simulink model "gm_rec_i2s"  (R2023b)
settings: Solver=VariableStepAuto  StartTime=0.0  StopTime=20  RelTol=1e-3
undefined symbols (not defined in the file or in its folder): cnt1_LRCLK, cnt2_SCLK
libraries: hdlsllib x4
(part 1 of 3)
settings Model: Creator=31651  LastModifiedBy=31651
settings DataIOCC: SignalLogging=off
settings OptimizationCC: BlockReduction=off  ConditionallyExecuteInputs=off  DefaultParameterBehavior=Inlined
settings DebuggingCC: AlgebraicLoopMsg=error  InheritedTsInSrcMsg=none
settings HardwareCC: ProdBitPerPointer=32  ProdBitPerSizeT=32  ProdBitPerPtrDiffT=32  ProdLargestAtomicFloat=None  ProdIntDivRoundTo=Undefined  ProdEndianess=Unspecified  ProdWordSize=32  ProdHWDeviceType=ASIC/FPGA->ASIC/FPGA  TargetBitPerPointer=64  TargetBitPerSizeT=64  TargetBitPerPtrDiffT=64  TargetLongLongMode=on  TargetIntDivRoundTo=Zero  TargetEndianess=LittleEndian  TargetWordSize=64  TargetHWDeviceType=Custom Processor->MATLAB Host Computer  ProdEqTarget=off

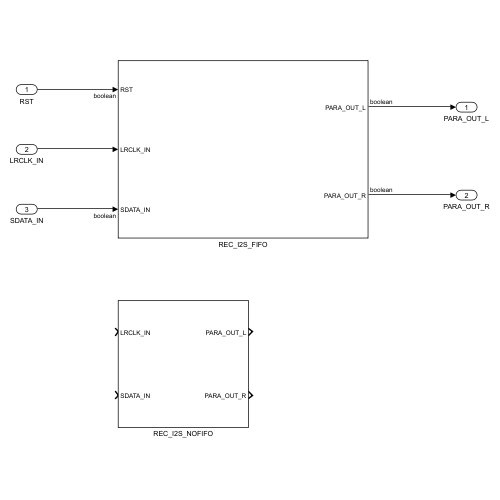
[thumbnail: Simulink's stored preview of the top-level diagram]
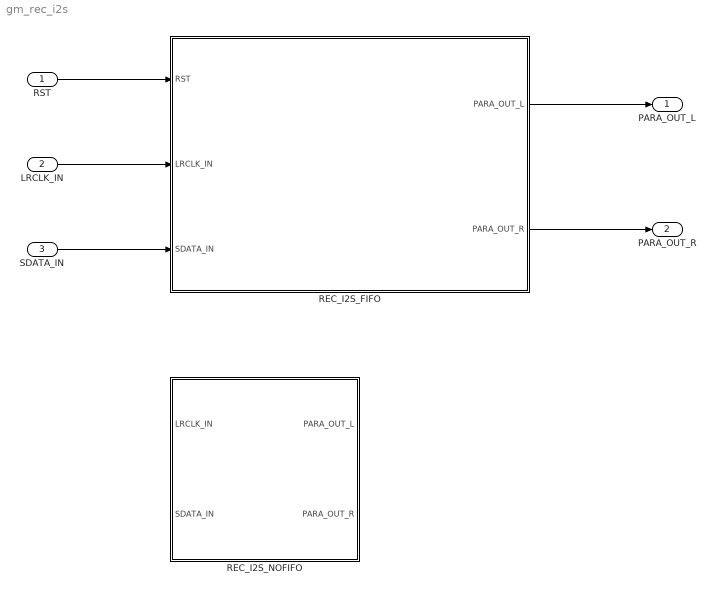
== system gm_rec_i2s ==
  RST : Inport
  LRCLK_IN : Inport  Port=2
  SDATA_IN : Inport  Port=3
  REC_I2S_FIFO : Subsystem
  REC_I2S_NOFIFO : Subsystem
  PARA_OUT_L : Outport
  PARA_OUT_R : Outport  Port=2
  wires:
  REC_I2S_FIFO/2(PARA_OUT_R) -> PARA_OUT_R/1
  REC_I2S_FIFO/1(PARA_OUT_L) -> PARA_OUT_L/1
  SDATA_IN/1 -> REC_I2S_FIFO/3(SDATA_IN)
  LRCLK_IN/1 -> REC_I2S_FIFO/2(LRCLK_IN)
  RST/1 -> REC_I2S_FIFO/1(RST)

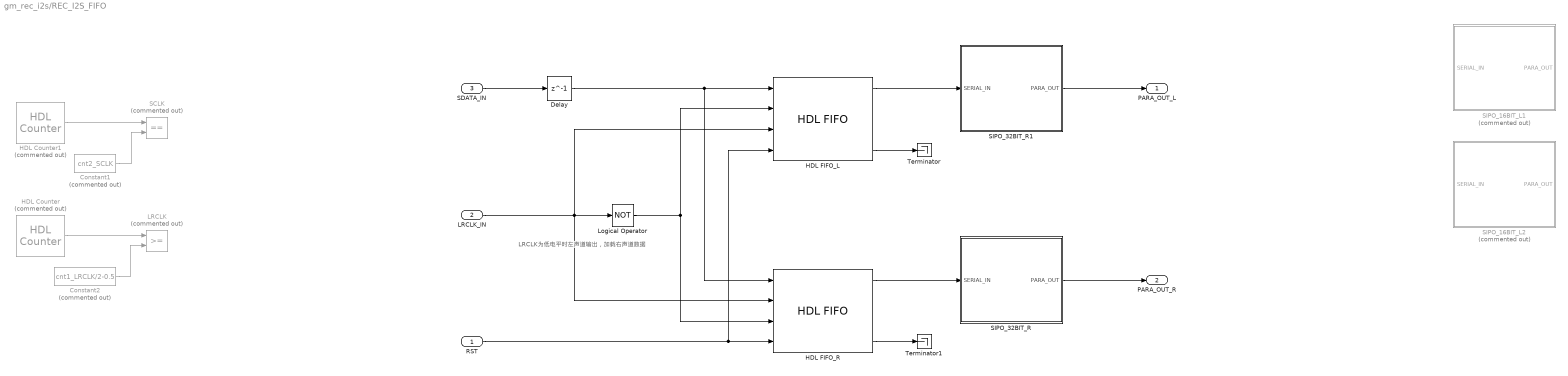
== system gm_rec_i2s/REC_I2S_FIFO ==
  note: LRCLK为低电平时左声道输出，加载右声道数据
  RST : Inport  OutDataTypeStr=boolean
  LRCLK_IN : Inport  Port=2
  SDATA_IN : Inport  Port=3  OutDataTypeStr=boolean
  Constant1 : Constant  Commented=on  Value=cnt2_SCLK  OutDataTypeStr=uint16
  Constant2 : Constant  Commented=on  Value=cnt1_LRCLK/2-0.5  OutDataTypeStr=uint16
  Delay : Delay  DelayLength=1  InitialCondition=0  SampleTime=1
  HDL Counter : hdlsllib/Sources/HDL Counter  Commented=on  CountType=Count limited  CountInit=0  CountStep=1  CountMax=cnt1_LRCLK  CountFromType=Initial value  CountFrom=0  CountResetPort=off  CountLoadPort=off  CountEnbPort=on  CountDirPort=off  CountHitOutputPort=off  CountDataType=Unsigned  CountWordLen=16  CountFracLen=0  CountSampTime=1
  HDL Counter1 : hdlsllib/Sources/HDL Counter  Commented=on  CountType=Count limited  CountInit=0  CountStep=1  CountMax=cnt2_SCLK  CountFromType=Initial value  CountFrom=0  CountResetPort=off  CountLoadPort=off  CountEnbPort=on  CountDirPort=off  CountHitOutputPort=off  CountDataType=Unsigned  CountWordLen=16  CountFracLen=0  CountSampTime=1
  HDL FIFO_L : hdlsllib/HDL RAMs/HDL FIFO  fifo_size=32  mode=Classic  ratio=1  push_msg=Warning  pop_msg=Warning  show_empty=on  show_full=on  show_num=on  LabelModeActiveChoice_Mode=Classic  rst_port=on
  HDL FIFO_R : hdlsllib/HDL RAMs/HDL FIFO  fifo_size=32  mode=Classic  ratio=1  push_msg=Warning  pop_msg=Warning  show_empty=on  show_full=on  show_num=on  LabelModeActiveChoice_Mode=Classic  rst_port=on
  LRCLK : RelationalOperator  Commented=on  OutDataTypeStr=boolean  InputSameDT=off
  Logical Operator : Logic  Operator=NOT  AllPortsSameDT=off  OutDataTypeStr=boolean
  SCLK : RelationalOperator  Commented=on  Operator===  OutDataTypeStr=boolean  InputSameDT=off
  SIPO_16BIT_L1 : Subsystem  Commented=on
  SIPO_16BIT_L2 : Subsystem  Commented=on
  SIPO_32BIT_R : Subsystem
  SIPO_32BIT_R1 : Subsystem
  Terminator : Terminator
  Terminator1 : Terminator
  PARA_OUT_L : Outport  OutDataTypeStr=boolean
  PARA_OUT_R : Outport  Port=2  OutDataTypeStr=boolean
  wires:
  HDL FIFO_L/1 -> SIPO_32BIT_R1/1(SERIAL_IN)
  HDL FIFO_R/1 -> SIPO_32BIT_R/1(SERIAL_IN)
  SIPO_32BIT_R/1(PARA_OUT) -> PARA_OUT_R/1
  SIPO_32BIT_R1/1(PARA_OUT) -> PARA_OUT_L/1
  RST/1 -> HDL FIFO_R/4, HDL FIFO_L/4
  Delay/1 -> HDL FIFO_L/1, HDL FIFO_R/1
  SDATA_IN/1 -> Delay/1
  HDL FIFO_R/4 -> Terminator1/1
  HDL FIFO_L/4 -> Terminator/1
  LRCLK_IN/1 -> Logical Operator/1, HDL FIFO_L/3, HDL FIFO_R/2
  Constant2/1 -> LRCLK/2
  Constant1/1 -> SCLK/2
  HDL Counter/1 -> LRCLK/1
  Logical Operator/1 -> HDL FIFO_R/3, HDL FIFO_L/2
  HDL Counter1/1 -> SCLK/1

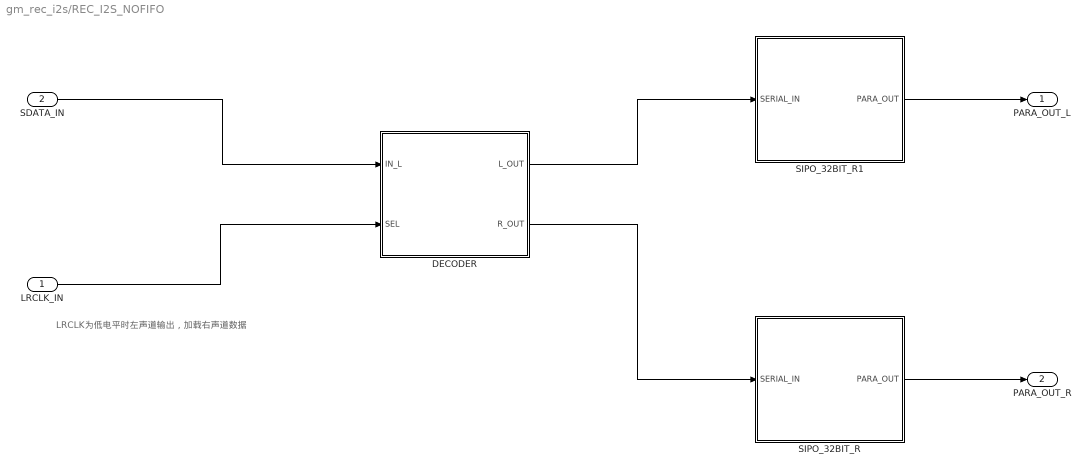
== system gm_rec_i2s/REC_I2S_NOFIFO ==
  note: LRCLK为低电平时左声道输出，加载右声道数据
  LRCLK_IN : Inport
  SDATA_IN : Inport  Port=2  OutDataTypeStr=boolean
  DECODER : Subsystem
  SIPO_32BIT_R : Subsystem
  SIPO_32BIT_R1 : Subsystem
  PARA_OUT_L : Outport  OutDataTypeStr=boolean
  PARA_OUT_R : Outport  Port=2  OutDataTypeStr=boolean
  wires:
  DECODER/2(R_OUT) -> SIPO_32BIT_R/1(SERIAL_IN)
  DECODER/1(L_OUT) -> SIPO_32BIT_R1/1(SERIAL_IN)
  LRCLK_IN/1 -> DECODER/2(SEL)
  SIPO_32BIT_R/1(PARA_OUT) -> PARA_OUT_R/1
  SDATA_IN/1 -> DECODER/1(IN_L)
  SIPO_32BIT_R1/1(PARA_OUT) -> PARA_OUT_L/1

== system gm_rec_i2s/REC_I2S_FIFO/SIPO_16BIT_L1 ==
  SERIAL_IN : Inport  OutDataTypeStr=boolean
  Merge : Merge
  SIPO_8BIT : Subsystem
  SIPO_8BIT1 : Subsystem
  Terminator : Terminator
  PARA_OUT : Outport  VectorParamsAs1DForOutWhenUnconnected=off
  wires:
  Merge/1 -> PARA_OUT/1
  SIPO_8BIT1/2(SERIAL_OUT) -> Terminator/1
  SIPO_8BIT1/1(PARA_OUT) -> Merge/1
  SIPO_8BIT/1(PARA_OUT) -> Merge/2
  SIPO_8BIT/2(SERIAL_OUT) -> SIPO_8BIT1/1(SERIAL_IN)
  SERIAL_IN/1 -> SIPO_8BIT/1(SERIAL_IN)

== system gm_rec_i2s/REC_I2S_FIFO/SIPO_16BIT_L2 ==
  SERIAL_IN : Inport  OutDataTypeStr=boolean
  Merge : Merge
  SIPO_8BIT : Subsystem
  SIPO_8BIT1 : Subsystem
  Terminator : Terminator
  PARA_OUT : Outport  VectorParamsAs1DForOutWhenUnconnected=off
  wires:
  Merge/1 -> PARA_OUT/1
  SIPO_8BIT1/2(SERIAL_OUT) -> Terminator/1
  SIPO_8BIT1/1(PARA_OUT) -> Merge/1
  SIPO_8BIT/1(PARA_OUT) -> Merge/2
  SIPO_8BIT/2(SERIAL_OUT) -> SIPO_8BIT1/1(SERIAL_IN)
  SERIAL_IN/1 -> SIPO_8BIT/1(SERIAL_IN)

== system gm_rec_i2s/REC_I2S_FIFO/SIPO_32BIT_R ==
  SERIAL_IN : Inport  OutDataTypeStr=boolean
  Subsystem : Subsystem
  PARA_OUT : Outport  OutDataTypeStr=boolean  VectorParamsAs1DForOutWhenUnconnected=off
  wires:
  Subsystem/1(PARA_OUT_32BIT) -> PARA_OUT/1
  SERIAL_IN/1 -> Subsystem/1(SERIAL_IN)

== system gm_rec_i2s/REC_I2S_FIFO/SIPO_32BIT_R1 ==
  SERIAL_IN : Inport  OutDataTypeStr=boolean
  Subsystem : Subsystem
  PARA_OUT : Outport  OutDataTypeStr=boolean  VectorParamsAs1DForOutWhenUnconnected=off
  wires:
  Subsystem/1(PARA_OUT_32BIT) -> PARA_OUT/1
  SERIAL_IN/1 -> Subsystem/1(SERIAL_IN)

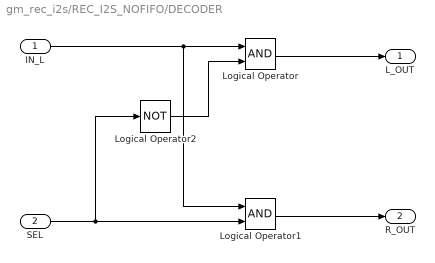
== system gm_rec_i2s/REC_I2S_NOFIFO/DECODER ==
  IN_L : Inport  OutDataTypeStr=boolean
  SEL : Inport  Port=2  OutDataTypeStr=boolean
  Logical Operator : Logic  AllPortsSameDT=off  OutDataTypeStr=boolean
  Logical Operator1 : Logic  AllPortsSameDT=off  OutDataTypeStr=boolean
  Logical Operator2 : Logic  Operator=NOT  AllPortsSameDT=off  OutDataTypeStr=boolean
  L_OUT : Outport  VectorParamsAs1DForOutWhenUnconnected=off
  R_OUT : Outport  Port=2  VectorParamsAs1DForOutWhenUnconnected=off
  wires:
  Logical Operator1/1 -> R_OUT/1
  Logical Operator/1 -> L_OUT/1
  IN_L/1 -> Logical Operator/1, Logical Operator1/1
  Logical Operator2/1 -> Logical Operator/2
  SEL/1 -> Logical Operator2/1, Logical Operator1/2

== system gm_rec_i2s/REC_I2S_NOFIFO/SIPO_32BIT_R ==
  SERIAL_IN : Inport  OutDataTypeStr=boolean
  Subsystem : Subsystem
  PARA_OUT : Outport  OutDataTypeStr=boolean  VectorParamsAs1DForOutWhenUnconnected=off
  wires:
  Subsystem/1(PARA_OUT_32BIT) -> PARA_OUT/1
  SERIAL_IN/1 -> Subsystem/1(SERIAL_IN)

== system gm_rec_i2s/REC_I2S_NOFIFO/SIPO_32BIT_R1 ==
  SERIAL_IN : Inport  OutDataTypeStr=boolean
  Subsystem : Subsystem
  PARA_OUT : Outport  OutDataTypeStr=boolean  VectorParamsAs1DForOutWhenUnconnected=off
  wires:
  Subsystem/1(PARA_OUT_32BIT) -> PARA_OUT/1
  SERIAL_IN/1 -> Subsystem/1(SERIAL_IN)

== system gm_rec_i2s/REC_I2S_FIFO/SIPO_16BIT_L1/SIPO_8BIT ==
  SERIAL_IN : Inport  OutDataTypeStr=boolean
  Merge : Merge
  SIPO_4BIT : Subsystem
  SIPO_4BIT1 : Subsystem
  PARA_OUT : Outport  VectorParamsAs1DForOutWhenUnconnected=off
  SERIAL_OUT : Outport  Port=2  VectorParamsAs1DForOutWhenUnconnected=off
  wires:
  SERIAL_IN/1 -> SIPO_4BIT/1(SERIAL_IN)
  SIPO_4BIT1/2(SERIAL_OUT) -> SERIAL_OUT/1
  SIPO_4BIT1/1(PARA_OUT) -> Merge/1
  SIPO_4BIT/2(SERIAL_OUT) -> SIPO_4BIT1/1(SERIAL_IN)
  Merge/1 -> PARA_OUT/1
  SIPO_4BIT/1(PARA_OUT) -> Merge/2

== system gm_rec_i2s/REC_I2S_FIFO/SIPO_16BIT_L1/SIPO_8BIT1 ==
  SERIAL_IN : Inport  OutDataTypeStr=boolean
  Merge : Merge
  SIPO_4BIT : Subsystem
  SIPO_4BIT1 : Subsystem
  PARA_OUT : Outport  VectorParamsAs1DForOutWhenUnconnected=off
  SERIAL_OUT : Outport  Port=2  VectorParamsAs1DForOutWhenUnconnected=off
  wires:
  SERIAL_IN/1 -> SIPO_4BIT/1(SERIAL_IN)
  SIPO_4BIT1/2(SERIAL_OUT) -> SERIAL_OUT/1
  SIPO_4BIT1/1(PARA_OUT) -> Merge/1
  SIPO_4BIT/2(SERIAL_OUT) -> SIPO_4BIT1/1(SERIAL_IN)
  Merge/1 -> PARA_OUT/1
  SIPO_4BIT/1(PARA_OUT) -> Merge/2

== system gm_rec_i2s/REC_I2S_FIFO/SIPO_16BIT_L2/SIPO_8BIT ==
  SERIAL_IN : Inport  OutDataTypeStr=boolean
  Merge : Merge
  SIPO_4BIT : Subsystem
  SIPO_4BIT1 : Subsystem
  PARA_OUT : Outport  VectorParamsAs1DForOutWhenUnconnected=off
  SERIAL_OUT : Outport  Port=2  VectorParamsAs1DForOutWhenUnconnected=off
  wires:
  SERIAL_IN/1 -> SIPO_4BIT/1(SERIAL_IN)
  SIPO_4BIT1/2(SERIAL_OUT) -> SERIAL_OUT/1
  SIPO_4BIT1/1(PARA_OUT) -> Merge/1
  SIPO_4BIT/2(SERIAL_OUT) -> SIPO_4BIT1/1(SERIAL_IN)
  Merge/1 -> PARA_OUT/1
  SIPO_4BIT/1(PARA_OUT) -> Merge/2

== system gm_rec_i2s/REC_I2S_FIFO/SIPO_16BIT_L2/SIPO_8BIT1 ==
  SERIAL_IN : Inport  OutDataTypeStr=boolean
  Merge : Merge
  SIPO_4BIT : Subsystem
  SIPO_4BIT1 : Subsystem
  PARA_OUT : Outport  VectorParamsAs1DForOutWhenUnconnected=off
  SERIAL_OUT : Outport  Port=2  VectorParamsAs1DForOutWhenUnconnected=off
  wires:
  SERIAL_IN/1 -> SIPO_4BIT/1(SERIAL_IN)
  SIPO_4BIT1/2(SERIAL_OUT) -> SERIAL_OUT/1
  SIPO_4BIT1/1(PARA_OUT) -> Merge/1
  SIPO_4BIT/2(SERIAL_OUT) -> SIPO_4BIT1/1(SERIAL_IN)
  Merge/1 -> PARA_OUT/1
  SIPO_4BIT/1(PARA_OUT) -> Merge/2

== system gm_rec_i2s/REC_I2S_FIFO/SIPO_32BIT_R/Subsystem ==
  SERIAL_IN : Inport  OutDataTypeStr=boolean
  SIPO_16BIT : Subsystem
  SIPO_16BIT1 : Subsystem
  Terminator : Terminator
  Vector Concatenate : Concatenate
  PARA_OUT_32BIT : Outport
  wires:
  Vector Concatenate/1 -> PARA_OUT_32BIT/1
  SIPO_16BIT1/2(SERIAL_OUT) -> Terminator/1
  SIPO_16BIT1/1(PARA_OUT) -> Vector Concatenate/1
  SIPO_16BIT/1(PARA_OUT) -> Vector Concatenate/2
  SIPO_16BIT/2(SERIAL_OUT) -> SIPO_16BIT1/1(SERIAL_IN)
  SERIAL_IN/1 -> SIPO_16BIT/1(SERIAL_IN)

== system gm_rec_i2s/REC_I2S_FIFO/SIPO_32BIT_R1/Subsystem ==
  SERIAL_IN : Inport  OutDataTypeStr=boolean
  SIPO_16BIT : Subsystem
  SIPO_16BIT1 : Subsystem
  Terminator : Terminator
  Vector Concatenate : Concatenate
  PARA_OUT_32BIT : Outport
  wires:
  Vector Concatenate/1 -> PARA_OUT_32BIT/1
  SIPO_16BIT1/2(SERIAL_OUT) -> Terminator/1
  SIPO_16BIT1/1(PARA_OUT) -> Vector Concatenate/1
  SIPO_16BIT/1(PARA_OUT) -> Vector Concatenate/2
  SIPO_16BIT/2(SERIAL_OUT) -> SIPO_16BIT1/1(SERIAL_IN)
  SERIAL_IN/1 -> SIPO_16BIT/1(SERIAL_IN)

== system gm_rec_i2s/REC_I2S_NOFIFO/SIPO_32BIT_R/Subsystem ==
  SERIAL_IN : Inport  OutDataTypeStr=boolean
  SIPO_16BIT : Subsystem
  SIPO_16BIT1 : Subsystem
  Terminator : Terminator
  Vector Concatenate : Concatenate
  PARA_OUT_32BIT : Outport
  wires:
  Vector Concatenate/1 -> PARA_OUT_32BIT/1
  SIPO_16BIT1/2(SERIAL_OUT) -> Terminator/1
  SIPO_16BIT1/1(PARA_OUT) -> Vector Concatenate/1
  SIPO_16BIT/1(PARA_OUT) -> Vector Concatenate/2
  SIPO_16BIT/2(SERIAL_OUT) -> SIPO_16BIT1/1(SERIAL_IN)
  SERIAL_IN/1 -> SIPO_16BIT/1(SERIAL_IN)

== system gm_rec_i2s/REC_I2S_NOFIFO/SIPO_32BIT_R1/Subsystem ==
  SERIAL_IN : Inport  OutDataTypeStr=boolean
  SIPO_16BIT : Subsystem
  SIPO_16BIT1 : Subsystem
  Terminator : Terminator
  Vector Concatenate : Concatenate
  PARA_OUT_32BIT : Outport
  wires:
  Vector Concatenate/1 -> PARA_OUT_32BIT/1
  SIPO_16BIT1/2(SERIAL_OUT) -> Terminator/1
  SIPO_16BIT1/1(PARA_OUT) -> Vector Concatenate/1
  SIPO_16BIT/1(PARA_OUT) -> Vector Concatenate/2
  SIPO_16BIT/2(SERIAL_OUT) -> SIPO_16BIT1/1(SERIAL_IN)
  SERIAL_IN/1 -> SIPO_16BIT/1(SERIAL_IN)

== system gm_rec_i2s/REC_I2S_FIFO/SIPO_16BIT_L1/SIPO_8BIT/SIPO_4BIT ==
  SERIAL_IN : Inport
  2BIT_SIPO : Subsystem
  2BIT_SIPO1 : Subsystem
  Merge : Merge
  PARA_OUT : Outport  VectorParamsAs1DForOutWhenUnconnected=off
  SERIAL_OUT : Outport  Port=2  VectorParamsAs1DForOutWhenUnconnected=off
  wires:
  2BIT_SIPO/2(SERIAL_OUT) -> 2BIT_SIPO1/1(SERIAL_IN)
  2BIT_SIPO1/1(PARA_OUT) -> Merge/1
  2BIT_SIPO/1(PARA_OUT) -> Merge/2
  Merge/1 -> PARA_OUT/1
  2BIT_SIPO1/2(SERIAL_OUT) -> SERIAL_OUT/1
  SERIAL_IN/1 -> 2BIT_SIPO/1(SERIAL_IN)

== system gm_rec_i2s/REC_I2S_FIFO/SIPO_16BIT_L1/SIPO_8BIT/SIPO_4BIT1 ==
  SERIAL_IN : Inport
  2BIT_SIPO : Subsystem
  2BIT_SIPO1 : Subsystem
  Merge : Merge
  PARA_OUT : Outport  VectorParamsAs1DForOutWhenUnconnected=off
  SERIAL_OUT : Outport  Port=2  VectorParamsAs1DForOutWhenUnconnected=off
  wires:
  2BIT_SIPO/2(SERIAL_OUT) -> 2BIT_SIPO1/1(SERIAL_IN)
  2BIT_SIPO1/1(PARA_OUT) -> Merge/1
  2BIT_SIPO/1(PARA_OUT) -> Merge/2
  Merge/1 -> PARA_OUT/1
  2BIT_SIPO1/2(SERIAL_OUT) -> SERIAL_OUT/1
  SERIAL_IN/1 -> 2BIT_SIPO/1(SERIAL_IN)

== system gm_rec_i2s/REC_I2S_FIFO/SIPO_16BIT_L1/SIPO_8BIT1/SIPO_4BIT ==
  SERIAL_IN : Inport
  2BIT_SIPO : Subsystem
  2BIT_SIPO1 : Subsystem
  Merge : Merge
  PARA_OUT : Outport  VectorParamsAs1DForOutWhenUnconnected=off
  SERIAL_OUT : Outport  Port=2  VectorParamsAs1DForOutWhenUnconnected=off
  wires:
  2BIT_SIPO/2(SERIAL_OUT) -> 2BIT_SIPO1/1(SERIAL_IN)
  2BIT_SIPO1/1(PARA_OUT) -> Merge/1
  2BIT_SIPO/1(PARA_OUT) -> Merge/2
  Merge/1 -> PARA_OUT/1
  2BIT_SIPO1/2(SERIAL_OUT) -> SERIAL_OUT/1
  SERIAL_IN/1 -> 2BIT_SIPO/1(SERIAL_IN)

== system gm_rec_i2s/REC_I2S_FIFO/SIPO_16BIT_L1/SIPO_8BIT1/SIPO_4BIT1 ==
  SERIAL_IN : Inport
  2BIT_SIPO : Subsystem
  2BIT_SIPO1 : Subsystem
  Merge : Merge
  PARA_OUT : Outport  VectorParamsAs1DForOutWhenUnconnected=off
  SERIAL_OUT : Outport  Port=2  VectorParamsAs1DForOutWhenUnconnected=off
  wires:
  2BIT_SIPO/2(SERIAL_OUT) -> 2BIT_SIPO1/1(SERIAL_IN)
  2BIT_SIPO1/1(PARA_OUT) -> Merge/1
  2BIT_SIPO/1(PARA_OUT) -> Merge/2
  Merge/1 -> PARA_OUT/1
  2BIT_SIPO1/2(SERIAL_OUT) -> SERIAL_OUT/1
  SERIAL_IN/1 -> 2BIT_SIPO/1(SERIAL_IN)

== system gm_rec_i2s/REC_I2S_FIFO/SIPO_16BIT_L2/SIPO_8BIT/SIPO_4BIT ==
  SERIAL_IN : Inport
  2BIT_SIPO : Subsystem
  2BIT_SIPO1 : Subsystem
  Merge : Merge
  PARA_OUT : Outport  VectorParamsAs1DForOutWhenUnconnected=off
  SERIAL_OUT : Outport  Port=2  VectorParamsAs1DForOutWhenUnconnected=off
  wires:
  2BIT_SIPO/2(SERIAL_OUT) -> 2BIT_SIPO1/1(SERIAL_IN)
  2BIT_SIPO1/1(PARA_OUT) -> Merge/1
  2BIT_SIPO/1(PARA_OUT) -> Merge/2
  Merge/1 -> PARA_OUT/1
  2BIT_SIPO1/2(SERIAL_OUT) -> SERIAL_OUT/1
  SERIAL_IN/1 -> 2BIT_SIPO/1(SERIAL_IN)

== system gm_rec_i2s/REC_I2S_FIFO/SIPO_16BIT_L2/SIPO_8BIT/SIPO_4BIT1 ==
  SERIAL_IN : Inport
  2BIT_SIPO : Subsystem
  2BIT_SIPO1 : Subsystem
  Merge : Merge
  PARA_OUT : Outport  VectorParamsAs1DForOutWhenUnconnected=off
  SERIAL_OUT : Outport  Port=2  VectorParamsAs1DForOutWhenUnconnected=off
  wires:
  2BIT_SIPO/2(SERIAL_OUT) -> 2BIT_SIPO1/1(SERIAL_IN)
  2BIT_SIPO1/1(PARA_OUT) -> Merge/1
  2BIT_SIPO/1(PARA_OUT) -> Merge/2
  Merge/1 -> PARA_OUT/1
  2BIT_SIPO1/2(SERIAL_OUT) -> SERIAL_OUT/1
  SERIAL_IN/1 -> 2BIT_SIPO/1(SERIAL_IN)

== system gm_rec_i2s/REC_I2S_FIFO/SIPO_16BIT_L2/SIPO_8BIT1/SIPO_4BIT ==
  SERIAL_IN : Inport
  2BIT_SIPO : Subsystem
  2BIT_SIPO1 : Subsystem
  Merge : Merge
  PARA_OUT : Outport  VectorParamsAs1DForOutWhenUnconnected=off
  SERIAL_OUT : Outport  Port=2  VectorParamsAs1DForOutWhenUnconnected=off
  wires:
  2BIT_SIPO/2(SERIAL_OUT) -> 2BIT_SIPO1/1(SERIAL_IN)
  2BIT_SIPO1/1(PARA_OUT) -> Merge/1
  2BIT_SIPO/1(PARA_OUT) -> Merge/2
  Merge/1 -> PARA_OUT/1
  2BIT_SIPO1/2(SERIAL_OUT) -> SERIAL_OUT/1
  SERIAL_IN/1 -> 2BIT_SIPO/1(SERIAL_IN)

== system gm_rec_i2s/REC_I2S_FIFO/SIPO_16BIT_L2/SIPO_8BIT1/SIPO_4BIT1 ==
  SERIAL_IN : Inport
  2BIT_SIPO : Subsystem
  2BIT_SIPO1 : Subsystem
  Merge : Merge
  PARA_OUT : Outport  VectorParamsAs1DForOutWhenUnconnected=off
  SERIAL_OUT : Outport  Port=2  VectorParamsAs1DForOutWhenUnconnected=off
  wires:
  2BIT_SIPO/2(SERIAL_OUT) -> 2BIT_SIPO1/1(SERIAL_IN)
  2BIT_SIPO1/1(PARA_OUT) -> Merge/1
  2BIT_SIPO/1(PARA_OUT) -> Merge/2
  Merge/1 -> PARA_OUT/1
  2BIT_SIPO1/2(SERIAL_OUT) -> SERIAL_OUT/1
  SERIAL_IN/1 -> 2BIT_SIPO/1(SERIAL_IN)

== system gm_rec_i2s/REC_I2S_FIFO/SIPO_32BIT_R/Subsystem/SIPO_16BIT ==
  SERIAL_IN : Inport  OutDataTypeStr=boolean
  SIPO_8BIT : Subsystem
  SIPO_8BIT1 : Subsystem
  Vector Concatenate : Concatenate
  PARA_OUT : Outport  OutDataTypeStr=boolean  VectorParamsAs1DForOutWhenUnconnected=off
  SERIAL_OUT : Outport  Port=2  OutDataTypeStr=boolean  VectorParamsAs1DForOutWhenUnconnected=off
  wires:
  SIPO_8BIT/1(PARA_OUT) -> Vector Concatenate/2
  SIPO_8BIT1/1(PARA_OUT) -> Vector Concatenate/1
  SIPO_8BIT1/2(SERIAL_OUT) -> SERIAL_OUT/1
  Vector Concatenate/1 -> PARA_OUT/1
  SERIAL_IN/1 -> SIPO_8BIT/1(SERIAL_IN)
  SIPO_8BIT/2(SERIAL_OUT) -> SIPO_8BIT1/1(SERIAL_IN)

== system gm_rec_i2s/REC_I2S_FIFO/SIPO_32BIT_R/Subsystem/SIPO_16BIT1 ==
  SERIAL_IN : Inport  OutDataTypeStr=boolean
  SIPO_8BIT : Subsystem
  SIPO_8BIT1 : Subsystem
  Vector Concatenate : Concatenate
  PARA_OUT : Outport  OutDataTypeStr=boolean  VectorParamsAs1DForOutWhenUnconnected=off
  SERIAL_OUT : Outport  Port=2  OutDataTypeStr=boolean  VectorParamsAs1DForOutWhenUnconnected=off
  wires:
  SIPO_8BIT/1(PARA_OUT) -> Vector Concatenate/2
  SIPO_8BIT1/1(PARA_OUT) -> Vector Concatenate/1
  SIPO_8BIT1/2(SERIAL_OUT) -> SERIAL_OUT/1
  Vector Concatenate/1 -> PARA_OUT/1
  SERIAL_IN/1 -> SIPO_8BIT/1(SERIAL_IN)
  SIPO_8BIT/2(SERIAL_OUT) -> SIPO_8BIT1/1(SERIAL_IN)

== system gm_rec_i2s/REC_I2S_FIFO/SIPO_32BIT_R1/Subsystem/SIPO_16BIT ==
  SERIAL_IN : Inport  OutDataTypeStr=boolean
  SIPO_8BIT : Subsystem
  SIPO_8BIT1 : Subsystem
  Vector Concatenate : Concatenate
  PARA_OUT : Outport  OutDataTypeStr=boolean  VectorParamsAs1DForOutWhenUnconnected=off
  SERIAL_OUT : Outport  Port=2  OutDataTypeStr=boolean  VectorParamsAs1DForOutWhenUnconnected=off
  wires:
  SIPO_8BIT/1(PARA_OUT) -> Vector Concatenate/2
  SIPO_8BIT1/1(PARA_OUT) -> Vector Concatenate/1
  SIPO_8BIT1/2(SERIAL_OUT) -> SERIAL_OUT/1
  Vector Concatenate/1 -> PARA_OUT/1
  SERIAL_IN/1 -> SIPO_8BIT/1(SERIAL_IN)
  SIPO_8BIT/2(SERIAL_OUT) -> SIPO_8BIT1/1(SERIAL_IN)

== system gm_rec_i2s/REC_I2S_FIFO/SIPO_32BIT_R1/Subsystem/SIPO_16BIT1 ==
  SERIAL_IN : Inport  OutDataTypeStr=boolean
  SIPO_8BIT : Subsystem
  SIPO_8BIT1 : Subsystem
  Vector Concatenate : Concatenate
  PARA_OUT : Outport  OutDataTypeStr=boolean  VectorParamsAs1DForOutWhenUnconnected=off
  SERIAL_OUT : Outport  Port=2  OutDataTypeStr=boolean  VectorParamsAs1DForOutWhenUnconnected=off
  wires:
  SIPO_8BIT/1(PARA_OUT) -> Vector Concatenate/2
  SIPO_8BIT1/1(PARA_OUT) -> Vector Concatenate/1
  SIPO_8BIT1/2(SERIAL_OUT) -> SERIAL_OUT/1
  Vector Concatenate/1 -> PARA_OUT/1
  SERIAL_IN/1 -> SIPO_8BIT/1(SERIAL_IN)
  SIPO_8BIT/2(SERIAL_OUT) -> SIPO_8BIT1/1(SERIAL_IN)

== system gm_rec_i2s/REC_I2S_NOFIFO/SIPO_32BIT_R/Subsystem/SIPO_16BIT ==
  SERIAL_IN : Inport  OutDataTypeStr=boolean
  SIPO_8BIT : Subsystem
  SIPO_8BIT1 : Subsystem
  Vector Concatenate : Concatenate
  PARA_OUT : Outport  OutDataTypeStr=boolean  VectorParamsAs1DForOutWhenUnconnected=off
  SERIAL_OUT : Outport  Port=2  OutDataTypeStr=boolean  VectorParamsAs1DForOutWhenUnconnected=off
  wires:
  SIPO_8BIT/1(PARA_OUT) -> Vector Concatenate/2
  SIPO_8BIT1/1(PARA_OUT) -> Vector Concatenate/1
  SIPO_8BIT1/2(SERIAL_OUT) -> SERIAL_OUT/1
  Vector Concatenate/1 -> PARA_OUT/1
  SERIAL_IN/1 -> SIPO_8BIT/1(SERIAL_IN)
  SIPO_8BIT/2(SERIAL_OUT) -> SIPO_8BIT1/1(SERIAL_IN)

== system gm_rec_i2s/REC_I2S_NOFIFO/SIPO_32BIT_R/Subsystem/SIPO_16BIT1 ==
  SERIAL_IN : Inport  OutDataTypeStr=boolean
  SIPO_8BIT : Subsystem
  SIPO_8BIT1 : Subsystem
  Vector Concatenate : Concatenate
  PARA_OUT : Outport  OutDataTypeStr=boolean  VectorParamsAs1DForOutWhenUnconnected=off
  SERIAL_OUT : Outport  Port=2  OutDataTypeStr=boolean  VectorParamsAs1DForOutWhenUnconnected=off
  wires:
  SIPO_8BIT/1(PARA_OUT) -> Vector Concatenate/2
  SIPO_8BIT1/1(PARA_OUT) -> Vector Concatenate/1
  SIPO_8BIT1/2(SERIAL_OUT) -> SERIAL_OUT/1
  Vector Concatenate/1 -> PARA_OUT/1
  SERIAL_IN/1 -> SIPO_8BIT/1(SERIAL_IN)
  SIPO_8BIT/2(SERIAL_OUT) -> SIPO_8BIT1/1(SERIAL_IN)

== system gm_rec_i2s/REC_I2S_NOFIFO/SIPO_32BIT_R1/Subsystem/SIPO_16BIT ==
  SERIAL_IN : Inport  OutDataTypeStr=boolean
  SIPO_8BIT : Subsystem
  SIPO_8BIT1 : Subsystem
  Vector Concatenate : Concatenate
  PARA_OUT : Outport  OutDataTypeStr=boolean  VectorParamsAs1DForOutWhenUnconnected=off
  SERIAL_OUT : Outport  Port=2  OutDataTypeStr=boolean  VectorParamsAs1DForOutWhenUnconnected=off
  wires:
  SIPO_8BIT/1(PARA_OUT) -> Vector Concatenate/2
  SIPO_8BIT1/1(PARA_OUT) -> Vector Concatenate/1
  SIPO_8BIT1/2(SERIAL_OUT) -> SERIAL_OUT/1
  Vector Concatenate/1 -> PARA_OUT/1
  SERIAL_IN/1 -> SIPO_8BIT/1(SERIAL_IN)
  SIPO_8BIT/2(SERIAL_OUT) -> SIPO_8BIT1/1(SERIAL_IN)

== system gm_rec_i2s/REC_I2S_NOFIFO/SIPO_32BIT_R1/Subsystem/SIPO_16BIT1 ==
  SERIAL_IN : Inport  OutDataTypeStr=boolean
  SIPO_8BIT : Subsystem
  SIPO_8BIT1 : Subsystem
  Vector Concatenate : Concatenate
  PARA_OUT : Outport  OutDataTypeStr=boolean  VectorParamsAs1DForOutWhenUnconnected=off
  SERIAL_OUT : Outport  Port=2  OutDataTypeStr=boolean  VectorParamsAs1DForOutWhenUnconnected=off
  wires:
  SIPO_8BIT/1(PARA_OUT) -> Vector Concatenate/2
  SIPO_8BIT1/1(PARA_OUT) -> Vector Concatenate/1
  SIPO_8BIT1/2(SERIAL_OUT) -> SERIAL_OUT/1
  Vector Concatenate/1 -> PARA_OUT/1
  SERIAL_IN/1 -> SIPO_8BIT/1(SERIAL_IN)
  SIPO_8BIT/2(SERIAL_OUT) -> SIPO_8BIT1/1(SERIAL_IN)

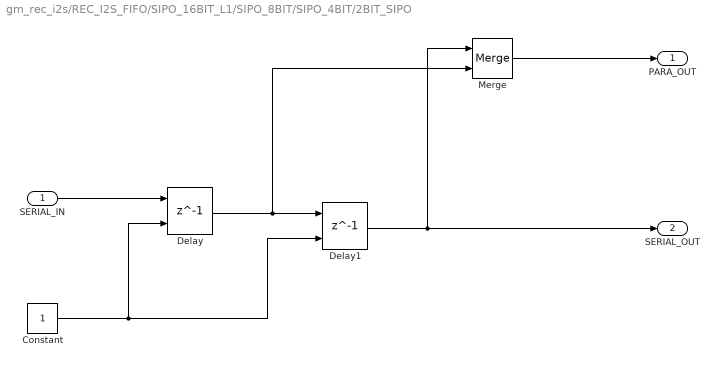
== system gm_rec_i2s/REC_I2S_FIFO/SIPO_16BIT_L1/SIPO_8BIT/SIPO_4BIT/2BIT_SIPO ==
  SERIAL_IN : Inport
  Constant : Constant  OutDataTypeStr=boolean  SampleTime=1
  Delay : Delay  DelayLength=1  InitialCondition=0  ShowEnablePort=on  SampleTime=1
      settings: InputPortMap=u0,e6
  Delay1 : Delay  DelayLength=1  InitialCondition=0  ShowEnablePort=on  SampleTime=1
      settings: InputPortMap=u0,e6
  Merge : Merge
  PARA_OUT : Outport  VectorParamsAs1DForOutWhenUnconnected=off
  SERIAL_OUT : Outport  Port=2  OutDataTypeStr=boolean  VectorParamsAs1DForOutWhenUnconnected=off
  wires:
  SERIAL_IN/1 -> Delay/1
  Delay1/1 -> SERIAL_OUT/1, Merge/1
  Merge/1 -> PARA_OUT/1
  Delay/1 -> Delay1/1, Merge/2
  Constant/1 -> Delay1/2, Delay/2

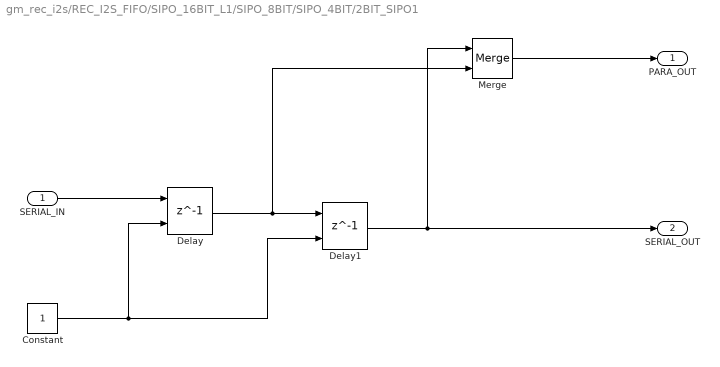
== system gm_rec_i2s/REC_I2S_FIFO/SIPO_16BIT_L1/SIPO_8BIT/SIPO_4BIT/2BIT_SIPO1 ==
  SERIAL_IN : Inport  OutDataTypeStr=boolean
  Constant : Constant  OutDataTypeStr=boolean  SampleTime=1
  Delay : Delay  DelayLength=1  InitialCondition=0  ShowEnablePort=on  SampleTime=1
      settings: InputPortMap=u0,e6
  Delay1 : Delay  DelayLength=1  InitialCondition=0  ShowEnablePort=on  SampleTime=1
      settings: InputPortMap=u0,e6
  Merge : Merge
  PARA_OUT : Outport  VectorParamsAs1DForOutWhenUnconnected=off
  SERIAL_OUT : Outport  Port=2  VectorParamsAs1DForOutWhenUnconnected=off
  wires:
  SERIAL_IN/1 -> Delay/1
  Delay1/1 -> SERIAL_OUT/1, Merge/1
  Merge/1 -> PARA_OUT/1
  Delay/1 -> Delay1/1, Merge/2
  Constant/1 -> Delay1/2, Delay/2

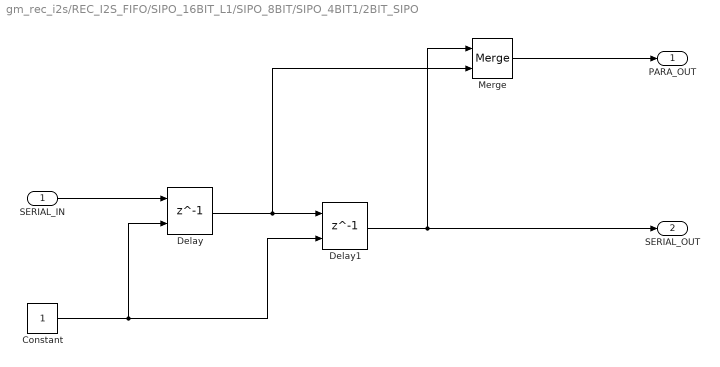
== system gm_rec_i2s/REC_I2S_FIFO/SIPO_16BIT_L1/SIPO_8BIT/SIPO_4BIT1/2BIT_SIPO ==
  SERIAL_IN : Inport
  Constant : Constant  OutDataTypeStr=boolean  SampleTime=1
  Delay : Delay  DelayLength=1  InitialCondition=0  ShowEnablePort=on  SampleTime=1
      settings: InputPortMap=u0,e6
  Delay1 : Delay  DelayLength=1  InitialCondition=0  ShowEnablePort=on  SampleTime=1
      settings: InputPortMap=u0,e6
  Merge : Merge
  PARA_OUT : Outport  VectorParamsAs1DForOutWhenUnconnected=off
  SERIAL_OUT : Outport  Port=2  VectorParamsAs1DForOutWhenUnconnected=off
  wires:
  SERIAL_IN/1 -> Delay/1
  Delay1/1 -> SERIAL_OUT/1, Merge/1
  Merge/1 -> PARA_OUT/1
  Delay/1 -> Delay1/1, Merge/2
  Constant/1 -> Delay1/2, Delay/2

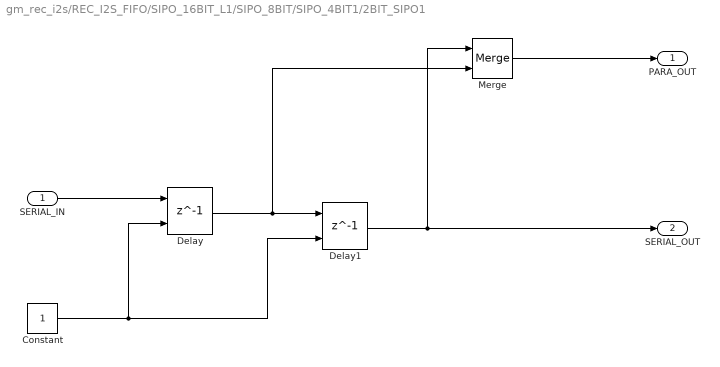
== system gm_rec_i2s/REC_I2S_FIFO/SIPO_16BIT_L1/SIPO_8BIT/SIPO_4BIT1/2BIT_SIPO1 ==
  SERIAL_IN : Inport
  Constant : Constant  OutDataTypeStr=boolean  SampleTime=1
  Delay : Delay  DelayLength=1  InitialCondition=0  ShowEnablePort=on  SampleTime=1
      settings: InputPortMap=u0,e6
  Delay1 : Delay  DelayLength=1  InitialCondition=0  ShowEnablePort=on  SampleTime=1
      settings: InputPortMap=u0,e6
  Merge : Merge
  PARA_OUT : Outport  VectorParamsAs1DForOutWhenUnconnected=off
  SERIAL_OUT : Outport  Port=2  VectorParamsAs1DForOutWhenUnconnected=off
  wires:
  SERIAL_IN/1 -> Delay/1
  Delay1/1 -> SERIAL_OUT/1, Merge/1
  Merge/1 -> PARA_OUT/1
  Delay/1 -> Delay1/1, Merge/2
  Constant/1 -> Delay1/2, Delay/2

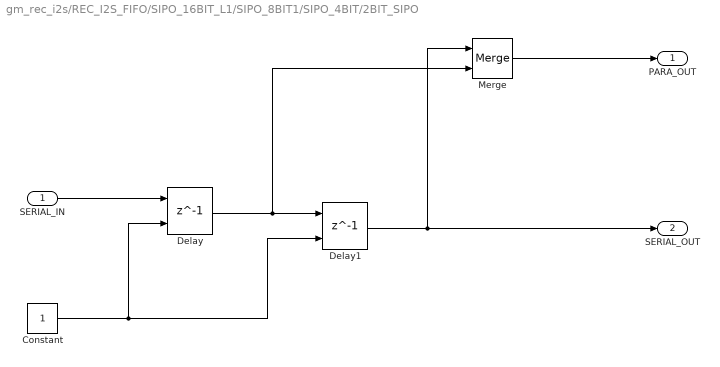
== system gm_rec_i2s/REC_I2S_FIFO/SIPO_16BIT_L1/SIPO_8BIT1/SIPO_4BIT/2BIT_SIPO ==
  SERIAL_IN : Inport
  Constant : Constant  OutDataTypeStr=boolean  SampleTime=1
  Delay : Delay  DelayLength=1  InitialCondition=0  ShowEnablePort=on  SampleTime=1
      settings: InputPortMap=u0,e6
  Delay1 : Delay  DelayLength=1  InitialCondition=0  ShowEnablePort=on  SampleTime=1
      settings: InputPortMap=u0,e6
  Merge : Merge
  PARA_OUT : Outport  VectorParamsAs1DForOutWhenUnconnected=off
  SERIAL_OUT : Outport  Port=2  OutDataTypeStr=boolean  VectorParamsAs1DForOutWhenUnconnected=off
  wires:
  SERIAL_IN/1 -> Delay/1
  Delay1/1 -> SERIAL_OUT/1, Merge/1
  Merge/1 -> PARA_OUT/1
  Delay/1 -> Delay1/1, Merge/2
  Constant/1 -> Delay1/2, Delay/2

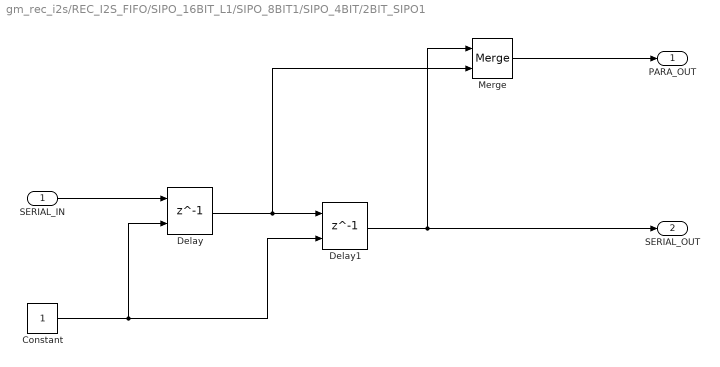
== system gm_rec_i2s/REC_I2S_FIFO/SIPO_16BIT_L1/SIPO_8BIT1/SIPO_4BIT/2BIT_SIPO1 ==
  SERIAL_IN : Inport  OutDataTypeStr=boolean
  Constant : Constant  OutDataTypeStr=boolean  SampleTime=1
  Delay : Delay  DelayLength=1  InitialCondition=0  ShowEnablePort=on  SampleTime=1
      settings: InputPortMap=u0,e6
  Delay1 : Delay  DelayLength=1  InitialCondition=0  ShowEnablePort=on  SampleTime=1
      settings: InputPortMap=u0,e6
  Merge : Merge
  PARA_OUT : Outport  VectorParamsAs1DForOutWhenUnconnected=off
  SERIAL_OUT : Outport  Port=2  VectorParamsAs1DForOutWhenUnconnected=off
  wires:
  SERIAL_IN/1 -> Delay/1
  Delay1/1 -> SERIAL_OUT/1, Merge/1
  Merge/1 -> PARA_OUT/1
  Delay/1 -> Delay1/1, Merge/2
  Constant/1 -> Delay1/2, Delay/2

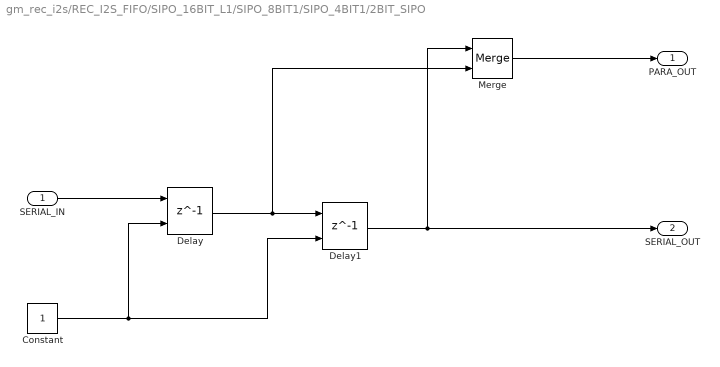
== system gm_rec_i2s/REC_I2S_FIFO/SIPO_16BIT_L1/SIPO_8BIT1/SIPO_4BIT1/2BIT_SIPO ==
  SERIAL_IN : Inport
  Constant : Constant  OutDataTypeStr=boolean  SampleTime=1
  Delay : Delay  DelayLength=1  InitialCondition=0  ShowEnablePort=on  SampleTime=1
      settings: InputPortMap=u0,e6
  Delay1 : Delay  DelayLength=1  InitialCondition=0  ShowEnablePort=on  SampleTime=1
      settings: InputPortMap=u0,e6
  Merge : Merge
  PARA_OUT : Outport  VectorParamsAs1DForOutWhenUnconnected=off
  SERIAL_OUT : Outport  Port=2  VectorParamsAs1DForOutWhenUnconnected=off
  wires:
  SERIAL_IN/1 -> Delay/1
  Delay1/1 -> SERIAL_OUT/1, Merge/1
  Merge/1 -> PARA_OUT/1
  Delay/1 -> Delay1/1, Merge/2
  Constant/1 -> Delay1/2, Delay/2

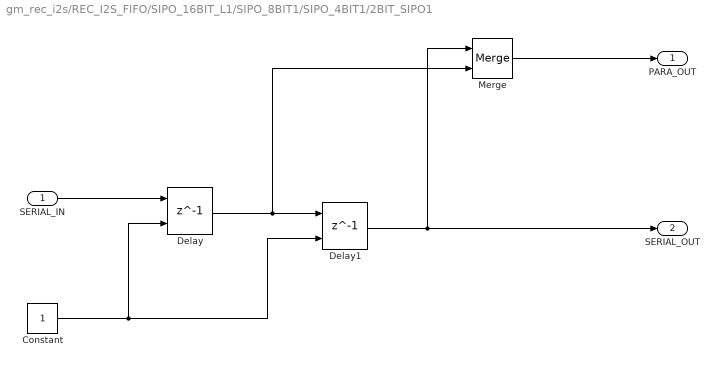
== system gm_rec_i2s/REC_I2S_FIFO/SIPO_16BIT_L1/SIPO_8BIT1/SIPO_4BIT1/2BIT_SIPO1 ==
  SERIAL_IN : Inport
  Constant : Constant  OutDataTypeStr=boolean  SampleTime=1
  Delay : Delay  DelayLength=1  InitialCondition=0  ShowEnablePort=on  SampleTime=1
      settings: InputPortMap=u0,e6
  Delay1 : Delay  DelayLength=1  InitialCondition=0  ShowEnablePort=on  SampleTime=1
      settings: InputPortMap=u0,e6
  Merge : Merge
  PARA_OUT : Outport  VectorParamsAs1DForOutWhenUnconnected=off
  SERIAL_OUT : Outport  Port=2  VectorParamsAs1DForOutWhenUnconnected=off
  wires:
  SERIAL_IN/1 -> Delay/1
  Delay1/1 -> SERIAL_OUT/1, Merge/1
  Merge/1 -> PARA_OUT/1
  Delay/1 -> Delay1/1, Merge/2
  Constant/1 -> Delay1/2, Delay/2

== system gm_rec_i2s/REC_I2S_FIFO/SIPO_16BIT_L2/SIPO_8BIT/SIPO_4BIT/2BIT_SIPO ==
  SERIAL_IN : Inport
  Constant : Constant  OutDataTypeStr=boolean  SampleTime=1
  Delay : Delay  DelayLength=1  InitialCondition=0  ShowEnablePort=on  SampleTime=1
      settings: InputPortMap=u0,e6
  Delay1 : Delay  DelayLength=1  InitialCondition=0  ShowEnablePort=on  SampleTime=1
      settings: InputPortMap=u0,e6
  Merge : Merge
  PARA_OUT : Outport  VectorParamsAs1DForOutWhenUnconnected=off
  SERIAL_OUT : Outport  Port=2  OutDataTypeStr=boolean  VectorParamsAs1DForOutWhenUnconnected=off
  wires:
  SERIAL_IN/1 -> Delay/1
  Delay1/1 -> SERIAL_OUT/1, Merge/1
  Merge/1 -> PARA_OUT/1
  Delay/1 -> Delay1/1, Merge/2
  Constant/1 -> Delay1/2, Delay/2

== system gm_rec_i2s/REC_I2S_FIFO/SIPO_16BIT_L2/SIPO_8BIT/SIPO_4BIT/2BIT_SIPO1 ==
  SERIAL_IN : Inport  OutDataTypeStr=boolean
  Constant : Constant  OutDataTypeStr=boolean  SampleTime=1
  Delay : Delay  DelayLength=1  InitialCondition=0  ShowEnablePort=on  SampleTime=1
      settings: InputPortMap=u0,e6
  Delay1 : Delay  DelayLength=1  InitialCondition=0  ShowEnablePort=on  SampleTime=1
      settings: InputPortMap=u0,e6
  Merge : Merge
  PARA_OUT : Outport  VectorParamsAs1DForOutWhenUnconnected=off
  SERIAL_OUT : Outport  Port=2  VectorParamsAs1DForOutWhenUnconnected=off
  wires:
  SERIAL_IN/1 -> Delay/1
  Delay1/1 -> SERIAL_OUT/1, Merge/1
  Merge/1 -> PARA_OUT/1
  Delay/1 -> Delay1/1, Merge/2
  Constant/1 -> Delay1/2, Delay/2

== system gm_rec_i2s/REC_I2S_FIFO/SIPO_16BIT_L2/SIPO_8BIT/SIPO_4BIT1/2BIT_SIPO ==
  SERIAL_IN : Inport
  Constant : Constant  OutDataTypeStr=boolean  SampleTime=1
  Delay : Delay  DelayLength=1  InitialCondition=0  ShowEnablePort=on  SampleTime=1
      settings: InputPortMap=u0,e6
  Delay1 : Delay  DelayLength=1  InitialCondition=0  ShowEnablePort=on  SampleTime=1
      settings: InputPortMap=u0,e6
  Merge : Merge
  PARA_OUT : Outport  VectorParamsAs1DForOutWhenUnconnected=off
  SERIAL_OUT : Outport  Port=2  VectorParamsAs1DForOutWhenUnconnected=off
  wires:
  SERIAL_IN/1 -> Delay/1
  Delay1/1 -> SERIAL_OUT/1, Merge/1
  Merge/1 -> PARA_OUT/1
  Delay/1 -> Delay1/1, Merge/2
  Constant/1 -> Delay1/2, Delay/2

== system gm_rec_i2s/REC_I2S_FIFO/SIPO_16BIT_L2/SIPO_8BIT/SIPO_4BIT1/2BIT_SIPO1 ==
  SERIAL_IN : Inport
  Constant : Constant  OutDataTypeStr=boolean  SampleTime=1
  Delay : Delay  DelayLength=1  InitialCondition=0  ShowEnablePort=on  SampleTime=1
      settings: InputPortMap=u0,e6
  Delay1 : Delay  DelayLength=1  InitialCondition=0  ShowEnablePort=on  SampleTime=1
      settings: InputPortMap=u0,e6
  Merge : Merge
  PARA_OUT : Outport  VectorParamsAs1DForOutWhenUnconnected=off
  SERIAL_OUT : Outport  Port=2  VectorParamsAs1DForOutWhenUnconnected=off
  wires:
  SERIAL_IN/1 -> Delay/1
  Delay1/1 -> SERIAL_OUT/1, Merge/1
  Merge/1 -> PARA_OUT/1
  Delay/1 -> Delay1/1, Merge/2
  Constant/1 -> Delay1/2, Delay/2

== system gm_rec_i2s/REC_I2S_FIFO/SIPO_16BIT_L2/SIPO_8BIT1/SIPO_4BIT/2BIT_SIPO ==
  SERIAL_IN : Inport
  Constant : Constant  OutDataTypeStr=boolean  SampleTime=1
  Delay : Delay  DelayLength=1  InitialCondition=0  ShowEnablePort=on  SampleTime=1
      settings: InputPortMap=u0,e6
  Delay1 : Delay  DelayLength=1  InitialCondition=0  ShowEnablePort=on  SampleTime=1
      settings: InputPortMap=u0,e6
  Merge : Merge
  PARA_OUT : Outport  VectorParamsAs1DForOutWhenUnconnected=off
  SERIAL_OUT : Outport  Port=2  OutDataTypeStr=boolean  VectorParamsAs1DForOutWhenUnconnected=off
  wires:
  SERIAL_IN/1 -> Delay/1
  Delay1/1 -> SERIAL_OUT/1, Merge/1
  Merge/1 -> PARA_OUT/1
  Delay/1 -> Delay1/1, Merge/2
  Constant/1 -> Delay1/2, Delay/2

== system gm_rec_i2s/REC_I2S_FIFO/SIPO_16BIT_L2/SIPO_8BIT1/SIPO_4BIT/2BIT_SIPO1 ==
  SERIAL_IN : Inport  OutDataTypeStr=boolean
  Constant : Constant  OutDataTypeStr=boolean  SampleTime=1
  Delay : Delay  DelayLength=1  InitialCondition=0  ShowEnablePort=on  SampleTime=1
      settings: InputPortMap=u0,e6
  Delay1 : Delay  DelayLength=1  InitialCondition=0  ShowEnablePort=on  SampleTime=1
      settings: InputPortMap=u0,e6
  Merge : Merge
  PARA_OUT : Outport  VectorParamsAs1DForOutWhenUnconnected=off
  SERIAL_OUT : Outport  Port=2  VectorParamsAs1DForOutWhenUnconnected=off
  wires:
  SERIAL_IN/1 -> Delay/1
  Delay1/1 -> SERIAL_OUT/1, Merge/1
  Merge/1 -> PARA_OUT/1
  Delay/1 -> Delay1/1, Merge/2
  Constant/1 -> Delay1/2, Delay/2

== system gm_rec_i2s/REC_I2S_FIFO/SIPO_16BIT_L2/SIPO_8BIT1/SIPO_4BIT1/2BIT_SIPO ==
  SERIAL_IN : Inport
  Constant : Constant  OutDataTypeStr=boolean  SampleTime=1
  Delay : Delay  DelayLength=1  InitialCondition=0  ShowEnablePort=on  SampleTime=1
      settings: InputPortMap=u0,e6
  Delay1 : Delay  DelayLength=1  InitialCondition=0  ShowEnablePort=on  SampleTime=1
      settings: InputPortMap=u0,e6
  Merge : Merge
  PARA_OUT : Outport  VectorParamsAs1DForOutWhenUnconnected=off
  SERIAL_OUT : Outport  Port=2  VectorParamsAs1DForOutWhenUnconnected=off
  wires:
  SERIAL_IN/1 -> Delay/1
  Delay1/1 -> SERIAL_OUT/1, Merge/1
  Merge/1 -> PARA_OUT/1
  Delay/1 -> Delay1/1, Merge/2
  Constant/1 -> Delay1/2, Delay/2

== system gm_rec_i2s/REC_I2S_FIFO/SIPO_16BIT_L2/SIPO_8BIT1/SIPO_4BIT1/2BIT_SIPO1 ==
  SERIAL_IN : Inport
  Constant : Constant  OutDataTypeStr=boolean  SampleTime=1
  Delay : Delay  DelayLength=1  InitialCondition=0  ShowEnablePort=on  SampleTime=1
      settings: InputPortMap=u0,e6
  Delay1 : Delay  DelayLength=1  InitialCondition=0  ShowEnablePort=on  SampleTime=1
      settings: InputPortMap=u0,e6
  Merge : Merge
  PARA_OUT : Outport  VectorParamsAs1DForOutWhenUnconnected=off
  SERIAL_OUT : Outport  Port=2  VectorParamsAs1DForOutWhenUnconnected=off
  wires:
  SERIAL_IN/1 -> Delay/1
  Delay1/1 -> SERIAL_OUT/1, Merge/1
  Merge/1 -> PARA_OUT/1
  Delay/1 -> Delay1/1, Merge/2
  Constant/1 -> Delay1/2, Delay/2

== system gm_rec_i2s/REC_I2S_FIFO/SIPO_32BIT_R/Subsystem/SIPO_16BIT/SIPO_8BIT ==
  SERIAL_IN : Inport  OutDataTypeStr=boolean
  SIPO_4BIT : Subsystem
  SIPO_4BIT1 : Subsystem
  Vector Concatenate : Concatenate
  PARA_OUT : Outport  VectorParamsAs1DForOutWhenUnconnected=off
  SERIAL_OUT : Outport  Port=2  VectorParamsAs1DForOutWhenUnconnected=off
  wires:
  SERIAL_IN/1 -> SIPO_4BIT/1(SERIAL_IN)
  SIPO_4BIT1/2(SERIAL_OUT) -> SERIAL_OUT/1
  SIPO_4BIT1/1(PARA_OUT) -> Vector Concatenate/1
  SIPO_4BIT/2(SERIAL_OUT) -> SIPO_4BIT1/1(SERIAL_IN)
  Vector Concatenate/1 -> PARA_OUT/1
  SIPO_4BIT/1(PARA_OUT) -> Vector Concatenate/2

== system gm_rec_i2s/REC_I2S_FIFO/SIPO_32BIT_R/Subsystem/SIPO_16BIT/SIPO_8BIT1 ==
  SERIAL_IN : Inport  OutDataTypeStr=boolean
  SIPO_4BIT : Subsystem
  SIPO_4BIT1 : Subsystem
  Vector Concatenate : Concatenate
  PARA_OUT : Outport  VectorParamsAs1DForOutWhenUnconnected=off
  SERIAL_OUT : Outport  Port=2  VectorParamsAs1DForOutWhenUnconnected=off
  wires:
  SERIAL_IN/1 -> SIPO_4BIT/1(SERIAL_IN)
  SIPO_4BIT1/2(SERIAL_OUT) -> SERIAL_OUT/1
  SIPO_4BIT1/1(PARA_OUT) -> Vector Concatenate/1
  SIPO_4BIT/2(SERIAL_OUT) -> SIPO_4BIT1/1(SERIAL_IN)
  Vector Concatenate/1 -> PARA_OUT/1
  SIPO_4BIT/1(PARA_OUT) -> Vector Concatenate/2

== system gm_rec_i2s/REC_I2S_FIFO/SIPO_32BIT_R/Subsystem/SIPO_16BIT1/SIPO_8BIT ==
  SERIAL_IN : Inport  OutDataTypeStr=boolean
  SIPO_4BIT : Subsystem
  SIPO_4BIT1 : Subsystem
  Vector Concatenate : Concatenate
  PARA_OUT : Outport  VectorParamsAs1DForOutWhenUnconnected=off
  SERIAL_OUT : Outport  Port=2  VectorParamsAs1DForOutWhenUnconnected=off
  wires:
  SERIAL_IN/1 -> SIPO_4BIT/1(SERIAL_IN)
  SIPO_4BIT1/2(SERIAL_OUT) -> SERIAL_OUT/1
  SIPO_4BIT1/1(PARA_OUT) -> Vector Concatenate/1
  SIPO_4BIT/2(SERIAL_OUT) -> SIPO_4BIT1/1(SERIAL_IN)
  Vector Concatenate/1 -> PARA_OUT/1
  SIPO_4BIT/1(PARA_OUT) -> Vector Concatenate/2

== system gm_rec_i2s/REC_I2S_FIFO/SIPO_32BIT_R/Subsystem/SIPO_16BIT1/SIPO_8BIT1 ==
  SERIAL_IN : Inport  OutDataTypeStr=boolean
  SIPO_4BIT : Subsystem
  SIPO_4BIT1 : Subsystem
  Vector Concatenate : Concatenate
  PARA_OUT : Outport  VectorParamsAs1DForOutWhenUnconnected=off
  SERIAL_OUT : Outport  Port=2  VectorParamsAs1DForOutWhenUnconnected=off
  wires:
  SERIAL_IN/1 -> SIPO_4BIT/1(SERIAL_IN)
  SIPO_4BIT1/2(SERIAL_OUT) -> SERIAL_OUT/1
  SIPO_4BIT1/1(PARA_OUT) -> Vector Concatenate/1
  SIPO_4BIT/2(SERIAL_OUT) -> SIPO_4BIT1/1(SERIAL_IN)
  Vector Concatenate/1 -> PARA_OUT/1
  SIPO_4BIT/1(PARA_OUT) -> Vector Concatenate/2

== system gm_rec_i2s/REC_I2S_FIFO/SIPO_32BIT_R1/Subsystem/SIPO_16BIT/SIPO_8BIT ==
  SERIAL_IN : Inport  OutDataTypeStr=boolean
  SIPO_4BIT : Subsystem
  SIPO_4BIT1 : Subsystem
  Vector Concatenate : Concatenate
  PARA_OUT : Outport  VectorParamsAs1DForOutWhenUnconnected=off
  SERIAL_OUT : Outport  Port=2  VectorParamsAs1DForOutWhenUnconnected=off
  wires:
  SERIAL_IN/1 -> SIPO_4BIT/1(SERIAL_IN)
  SIPO_4BIT1/2(SERIAL_OUT) -> SERIAL_OUT/1
  SIPO_4BIT1/1(PARA_OUT) -> Vector Concatenate/1
  SIPO_4BIT/2(SERIAL_OUT) -> SIPO_4BIT1/1(SERIAL_IN)
  Vector Concatenate/1 -> PARA_OUT/1
  SIPO_4BIT/1(PARA_OUT) -> Vector Concatenate/2

== system gm_rec_i2s/REC_I2S_FIFO/SIPO_32BIT_R1/Subsystem/SIPO_16BIT/SIPO_8BIT1 ==
  SERIAL_IN : Inport  OutDataTypeStr=boolean
  SIPO_4BIT : Subsystem
  SIPO_4BIT1 : Subsystem
  Vector Concatenate : Concatenate
  PARA_OUT : Outport  VectorParamsAs1DForOutWhenUnconnected=off
  SERIAL_OUT : Outport  Port=2  VectorParamsAs1DForOutWhenUnconnected=off
  wires:
  SERIAL_IN/1 -> SIPO_4BIT/1(SERIAL_IN)
  SIPO_4BIT1/2(SERIAL_OUT) -> SERIAL_OUT/1
  SIPO_4BIT1/1(PARA_OUT) -> Vector Concatenate/1
  SIPO_4BIT/2(SERIAL_OUT) -> SIPO_4BIT1/1(SERIAL_IN)
  Vector Concatenate/1 -> PARA_OUT/1
  SIPO_4BIT/1(PARA_OUT) -> Vector Concatenate/2

== system gm_rec_i2s/REC_I2S_FIFO/SIPO_32BIT_R1/Subsystem/SIPO_16BIT1/SIPO_8BIT ==
  SERIAL_IN : Inport  OutDataTypeStr=boolean
  SIPO_4BIT : Subsystem
  SIPO_4BIT1 : Subsystem
  Vector Concatenate : Concatenate
  PARA_OUT : Outport  VectorParamsAs1DForOutWhenUnconnected=off
  SERIAL_OUT : Outport  Port=2  VectorParamsAs1DForOutWhenUnconnected=off
  wires:
  SERIAL_IN/1 -> SIPO_4BIT/1(SERIAL_IN)
  SIPO_4BIT1/2(SERIAL_OUT) -> SERIAL_OUT/1
  SIPO_4BIT1/1(PARA_OUT) -> Vector Concatenate/1
  SIPO_4BIT/2(SERIAL_OUT) -> SIPO_4BIT1/1(SERIAL_IN)
  Vector Concatenate/1 -> PARA_OUT/1
  SIPO_4BIT/1(PARA_OUT) -> Vector Concatenate/2

== system gm_rec_i2s/REC_I2S_FIFO/SIPO_32BIT_R1/Subsystem/SIPO_16BIT1/SIPO_8BIT1 ==
  SERIAL_IN : Inport  OutDataTypeStr=boolean
  SIPO_4BIT : Subsystem
  SIPO_4BIT1 : Subsystem
  Vector Concatenate : Concatenate
  PARA_OUT : Outport  VectorParamsAs1DForOutWhenUnconnected=off
  SERIAL_OUT : Outport  Port=2  VectorParamsAs1DForOutWhenUnconnected=off
  wires:
  SERIAL_IN/1 -> SIPO_4BIT/1(SERIAL_IN)
  SIPO_4BIT1/2(SERIAL_OUT) -> SERIAL_OUT/1
  SIPO_4BIT1/1(PARA_OUT) -> Vector Concatenate/1
  SIPO_4BIT/2(SERIAL_OUT) -> SIPO_4BIT1/1(SERIAL_IN)
  Vector Concatenate/1 -> PARA_OUT/1
  SIPO_4BIT/1(PARA_OUT) -> Vector Concatenate/2

== system gm_rec_i2s/REC_I2S_NOFIFO/SIPO_32BIT_R/Subsystem/SIPO_16BIT/SIPO_8BIT ==
  SERIAL_IN : Inport  OutDataTypeStr=boolean
  SIPO_4BIT : Subsystem
  SIPO_4BIT1 : Subsystem
  Vector Concatenate : Concatenate
  PARA_OUT : Outport  VectorParamsAs1DForOutWhenUnconnected=off
  SERIAL_OUT : Outport  Port=2  VectorParamsAs1DForOutWhenUnconnected=off
  wires:
  SERIAL_IN/1 -> SIPO_4BIT/1(SERIAL_IN)
  SIPO_4BIT1/2(SERIAL_OUT) -> SERIAL_OUT/1
  SIPO_4BIT1/1(PARA_OUT) -> Vector Concatenate/1
  SIPO_4BIT/2(SERIAL_OUT) -> SIPO_4BIT1/1(SERIAL_IN)
  Vector Concatenate/1 -> PARA_OUT/1
  SIPO_4BIT/1(PARA_OUT) -> Vector Concatenate/2

== system gm_rec_i2s/REC_I2S_NOFIFO/SIPO_32BIT_R/Subsystem/SIPO_16BIT/SIPO_8BIT1 ==
  SERIAL_IN : Inport  OutDataTypeStr=boolean
  SIPO_4BIT : Subsystem
  SIPO_4BIT1 : Subsystem
  Vector Concatenate : Concatenate
  PARA_OUT : Outport  VectorParamsAs1DForOutWhenUnconnected=off
  SERIAL_OUT : Outport  Port=2  VectorParamsAs1DForOutWhenUnconnected=off
  wires:
  SERIAL_IN/1 -> SIPO_4BIT/1(SERIAL_IN)
  SIPO_4BIT1/2(SERIAL_OUT) -> SERIAL_OUT/1
  SIPO_4BIT1/1(PARA_OUT) -> Vector Concatenate/1
  SIPO_4BIT/2(SERIAL_OUT) -> SIPO_4BIT1/1(SERIAL_IN)
  Vector Concatenate/1 -> PARA_OUT/1
  SIPO_4BIT/1(PARA_OUT) -> Vector Concatenate/2

== system gm_rec_i2s/REC_I2S_NOFIFO/SIPO_32BIT_R/Subsystem/SIPO_16BIT1/SIPO_8BIT ==
  SERIAL_IN : Inport  OutDataTypeStr=boolean
  SIPO_4BIT : Subsystem
  SIPO_4BIT1 : Subsystem
  Vector Concatenate : Concatenate
  PARA_OUT : Outport  VectorParamsAs1DForOutWhenUnconnected=off
  SERIAL_OUT : Outport  Port=2  VectorParamsAs1DForOutWhenUnconnected=off
  wires:
  SERIAL_IN/1 -> SIPO_4BIT/1(SERIAL_IN)
  SIPO_4BIT1/2(SERIAL_OUT) -> SERIAL_OUT/1
  SIPO_4BIT1/1(PARA_OUT) -> Vector Concatenate/1
  SIPO_4BIT/2(SERIAL_OUT) -> SIPO_4BIT1/1(SERIAL_IN)
  Vector Concatenate/1 -> PARA_OUT/1
  SIPO_4BIT/1(PARA_OUT) -> Vector Concatenate/2

== system gm_rec_i2s/REC_I2S_NOFIFO/SIPO_32BIT_R/Subsystem/SIPO_16BIT1/SIPO_8BIT1 ==
  SERIAL_IN : Inport  OutDataTypeStr=boolean
  SIPO_4BIT : Subsystem
  SIPO_4BIT1 : Subsystem
  Vector Concatenate : Concatenate
  PARA_OUT : Outport  VectorParamsAs1DForOutWhenUnconnected=off
  SERIAL_OUT : Outport  Port=2  VectorParamsAs1DForOutWhenUnconnected=off
  wires:
  SERIAL_IN/1 -> SIPO_4BIT/1(SERIAL_IN)
  SIPO_4BIT1/2(SERIAL_OUT) -> SERIAL_OUT/1
  SIPO_4BIT1/1(PARA_OUT) -> Vector Concatenate/1
  SIPO_4BIT/2(SERIAL_OUT) -> SIPO_4BIT1/1(SERIAL_IN)
  Vector Concatenate/1 -> PARA_OUT/1
  SIPO_4BIT/1(PARA_OUT) -> Vector Concatenate/2

== system gm_rec_i2s/REC_I2S_NOFIFO/SIPO_32BIT_R1/Subsystem/SIPO_16BIT/SIPO_8BIT ==
  SERIAL_IN : Inport  OutDataTypeStr=boolean
  SIPO_4BIT : Subsystem
  SIPO_4BIT1 : Subsystem
  Vector Concatenate : Concatenate
  PARA_OUT : Outport  VectorParamsAs1DForOutWhenUnconnected=off
  SERIAL_OUT : Outport  Port=2  VectorParamsAs1DForOutWhenUnconnected=off
  wires:
  SERIAL_IN/1 -> SIPO_4BIT/1(SERIAL_IN)
  SIPO_4BIT1/2(SERIAL_OUT) -> SERIAL_OUT/1
  SIPO_4BIT1/1(PARA_OUT) -> Vector Concatenate/1
  SIPO_4BIT/2(SERIAL_OUT) -> SIPO_4BIT1/1(SERIAL_IN)
  Vector Concatenate/1 -> PARA_OUT/1
  SIPO_4BIT/1(PARA_OUT) -> Vector Concatenate/2

== system gm_rec_i2s/REC_I2S_NOFIFO/SIPO_32BIT_R1/Subsystem/SIPO_16BIT/SIPO_8BIT1 ==
  SERIAL_IN : Inport  OutDataTypeStr=boolean
  SIPO_4BIT : Subsystem
  SIPO_4BIT1 : Subsystem
  Vector Concatenate : Concatenate
  PARA_OUT : Outport  VectorParamsAs1DForOutWhenUnconnected=off
  SERIAL_OUT : Outport  Port=2  VectorParamsAs1DForOutWhenUnconnected=off
  wires:
  SERIAL_IN/1 -> SIPO_4BIT/1(SERIAL_IN)
  SIPO_4BIT1/2(SERIAL_OUT) -> SERIAL_OUT/1
  SIPO_4BIT1/1(PARA_OUT) -> Vector Concatenate/1
  SIPO_4BIT/2(SERIAL_OUT) -> SIPO_4BIT1/1(SERIAL_IN)
  Vector Concatenate/1 -> PARA_OUT/1
  SIPO_4BIT/1(PARA_OUT) -> Vector Concatenate/2

== system gm_rec_i2s/REC_I2S_NOFIFO/SIPO_32BIT_R1/Subsystem/SIPO_16BIT1/SIPO_8BIT ==
  SERIAL_IN : Inport  OutDataTypeStr=boolean
  SIPO_4BIT : Subsystem
  SIPO_4BIT1 : Subsystem
  Vector Concatenate : Concatenate
  PARA_OUT : Outport  VectorParamsAs1DForOutWhenUnconnected=off
  SERIAL_OUT : Outport  Port=2  VectorParamsAs1DForOutWhenUnconnected=off
  wires:
  SERIAL_IN/1 -> SIPO_4BIT/1(SERIAL_IN)
  SIPO_4BIT1/2(SERIAL_OUT) -> SERIAL_OUT/1
  SIPO_4BIT1/1(PARA_OUT) -> Vector Concatenate/1
  SIPO_4BIT/2(SERIAL_OUT) -> SIPO_4BIT1/1(SERIAL_IN)
  Vector Concatenate/1 -> PARA_OUT/1
  SIPO_4BIT/1(PARA_OUT) -> Vector Concatenate/2

== system gm_rec_i2s/REC_I2S_NOFIFO/SIPO_32BIT_R1/Subsystem/SIPO_16BIT1/SIPO_8BIT1 ==
  SERIAL_IN : Inport  OutDataTypeStr=boolean
  SIPO_4BIT : Subsystem
  SIPO_4BIT1 : Subsystem
  Vector Concatenate : Concatenate
  PARA_OUT : Outport  VectorParamsAs1DForOutWhenUnconnected=off
  SERIAL_OUT : Outport  Port=2  VectorParamsAs1DForOutWhenUnconnected=off
  wires:
  SERIAL_IN/1 -> SIPO_4BIT/1(SERIAL_IN)
  SIPO_4BIT1/2(SERIAL_OUT) -> SERIAL_OUT/1
  SIPO_4BIT1/1(PARA_OUT) -> Vector Concatenate/1
  SIPO_4BIT/2(SERIAL_OUT) -> SIPO_4BIT1/1(SERIAL_IN)
  Vector Concatenate/1 -> PARA_OUT/1
  SIPO_4BIT/1(PARA_OUT) -> Vector Concatenate/2

== system gm_rec_i2s/REC_I2S_FIFO/SIPO_32BIT_R/Subsystem/SIPO_16BIT/SIPO_8BIT/SIPO_4BIT ==
  SERIAL_IN : Inport
  2BIT_SIPO : Subsystem
  2BIT_SIPO1 : Subsystem
  Vector Concatenate : Concatenate
  PARA_OUT : Outport  VectorParamsAs1DForOutWhenUnconnected=off
  SERIAL_OUT : Outport  Port=2  VectorParamsAs1DForOutWhenUnconnected=off
  wires:
  2BIT_SIPO/2(SERIAL_OUT) -> 2BIT_SIPO1/1(SERIAL_IN)
  2BIT_SIPO1/1(PARA_OUT) -> Vector Concatenate/1
  2BIT_SIPO/1(PARA_OUT) -> Vector Concatenate/2
  Vector Concatenate/1 -> PARA_OUT/1
  2BIT_SIPO1/2(SERIAL_OUT) -> SERIAL_OUT/1
  SERIAL_IN/1 -> 2BIT_SIPO/1(SERIAL_IN)

== system gm_rec_i2s/REC_I2S_FIFO/SIPO_32BIT_R/Subsystem/SIPO_16BIT/SIPO_8BIT/SIPO_4BIT1 ==
  SERIAL_IN : Inport
  2BIT_SIPO : Subsystem
  2BIT_SIPO1 : Subsystem
  Vector Concatenate : Concatenate
  PARA_OUT : Outport  VectorParamsAs1DForOutWhenUnconnected=off
  SERIAL_OUT : Outport  Port=2  VectorParamsAs1DForOutWhenUnconnected=off
  wires:
  2BIT_SIPO/2(SERIAL_OUT) -> 2BIT_SIPO1/1(SERIAL_IN)
  2BIT_SIPO1/1(PARA_OUT) -> Vector Concatenate/1
  2BIT_SIPO/1(PARA_OUT) -> Vector Concatenate/2
  Vector Concatenate/1 -> PARA_OUT/1
  2BIT_SIPO1/2(SERIAL_OUT) -> SERIAL_OUT/1
  SERIAL_IN/1 -> 2BIT_SIPO/1(SERIAL_IN)

== system gm_rec_i2s/REC_I2S_FIFO/SIPO_32BIT_R/Subsystem/SIPO_16BIT/SIPO_8BIT1/SIPO_4BIT ==
  SERIAL_IN : Inport
  2BIT_SIPO : Subsystem
  2BIT_SIPO1 : Subsystem
  Vector Concatenate : Concatenate
  PARA_OUT : Outport  VectorParamsAs1DForOutWhenUnconnected=off
  SERIAL_OUT : Outport  Port=2  VectorParamsAs1DForOutWhenUnconnected=off
  wires:
  2BIT_SIPO/2(SERIAL_OUT) -> 2BIT_SIPO1/1(SERIAL_IN)
  2BIT_SIPO1/1(PARA_OUT) -> Vector Concatenate/1
  2BIT_SIPO/1(PARA_OUT) -> Vector Concatenate/2
  Vector Concatenate/1 -> PARA_OUT/1
  2BIT_SIPO1/2(SERIAL_OUT) -> SERIAL_OUT/1
  SERIAL_IN/1 -> 2BIT_SIPO/1(SERIAL_IN)

== system gm_rec_i2s/REC_I2S_FIFO/SIPO_32BIT_R/Subsystem/SIPO_16BIT/SIPO_8BIT1/SIPO_4BIT1 ==
  SERIAL_IN : Inport
  2BIT_SIPO : Subsystem
  2BIT_SIPO1 : Subsystem
  Vector Concatenate : Concatenate
  PARA_OUT : Outport  VectorParamsAs1DForOutWhenUnconnected=off
  SERIAL_OUT : Outport  Port=2  VectorParamsAs1DForOutWhenUnconnected=off
  wires:
  2BIT_SIPO/2(SERIAL_OUT) -> 2BIT_SIPO1/1(SERIAL_IN)
  2BIT_SIPO1/1(PARA_OUT) -> Vector Concatenate/1
  2BIT_SIPO/1(PARA_OUT) -> Vector Concatenate/2
  Vector Concatenate/1 -> PARA_OUT/1
  2BIT_SIPO1/2(SERIAL_OUT) -> SERIAL_OUT/1
  SERIAL_IN/1 -> 2BIT_SIPO/1(SERIAL_IN)

== system gm_rec_i2s/REC_I2S_FIFO/SIPO_32BIT_R/Subsystem/SIPO_16BIT1/SIPO_8BIT/SIPO_4BIT ==
  SERIAL_IN : Inport
  2BIT_SIPO : Subsystem
  2BIT_SIPO1 : Subsystem
  Vector Concatenate : Concatenate
  PARA_OUT : Outport  VectorParamsAs1DForOutWhenUnconnected=off
  SERIAL_OUT : Outport  Port=2  VectorParamsAs1DForOutWhenUnconnected=off
  wires:
  2BIT_SIPO/2(SERIAL_OUT) -> 2BIT_SIPO1/1(SERIAL_IN)
  2BIT_SIPO1/1(PARA_OUT) -> Vector Concatenate/1
  2BIT_SIPO/1(PARA_OUT) -> Vector Concatenate/2
  Vector Concatenate/1 -> PARA_OUT/1
  2BIT_SIPO1/2(SERIAL_OUT) -> SERIAL_OUT/1
  SERIAL_IN/1 -> 2BIT_SIPO/1(SERIAL_IN)

== system gm_rec_i2s/REC_I2S_FIFO/SIPO_32BIT_R/Subsystem/SIPO_16BIT1/SIPO_8BIT/SIPO_4BIT1 ==
  SERIAL_IN : Inport
  2BIT_SIPO : Subsystem
  2BIT_SIPO1 : Subsystem
  Vector Concatenate : Concatenate
  PARA_OUT : Outport  VectorParamsAs1DForOutWhenUnconnected=off
  SERIAL_OUT : Outport  Port=2  VectorParamsAs1DForOutWhenUnconnected=off
  wires:
  2BIT_SIPO/2(SERIAL_OUT) -> 2BIT_SIPO1/1(SERIAL_IN)
  2BIT_SIPO1/1(PARA_OUT) -> Vector Concatenate/1
  2BIT_SIPO/1(PARA_OUT) -> Vector Concatenate/2
  Vector Concatenate/1 -> PARA_OUT/1
  2BIT_SIPO1/2(SERIAL_OUT) -> SERIAL_OUT/1
  SERIAL_IN/1 -> 2BIT_SIPO/1(SERIAL_IN)

== system gm_rec_i2s/REC_I2S_FIFO/SIPO_32BIT_R/Subsystem/SIPO_16BIT1/SIPO_8BIT1/SIPO_4BIT ==
  SERIAL_IN : Inport
  2BIT_SIPO : Subsystem
  2BIT_SIPO1 : Subsystem
  Vector Concatenate : Concatenate
  PARA_OUT : Outport  VectorParamsAs1DForOutWhenUnconnected=off
  SERIAL_OUT : Outport  Port=2  VectorParamsAs1DForOutWhenUnconnected=off
  wires:
  2BIT_SIPO/2(SERIAL_OUT) -> 2BIT_SIPO1/1(SERIAL_IN)
  2BIT_SIPO1/1(PARA_OUT) -> Vector Concatenate/1
  2BIT_SIPO/1(PARA_OUT) -> Vector Concatenate/2
  Vector Concatenate/1 -> PARA_OUT/1
  2BIT_SIPO1/2(SERIAL_OUT) -> SERIAL_OUT/1
  SERIAL_IN/1 -> 2BIT_SIPO/1(SERIAL_IN)

== system gm_rec_i2s/REC_I2S_FIFO/SIPO_32BIT_R/Subsystem/SIPO_16BIT1/SIPO_8BIT1/SIPO_4BIT1 ==
  SERIAL_IN : Inport
  2BIT_SIPO : Subsystem
  2BIT_SIPO1 : Subsystem
  Vector Concatenate : Concatenate
  PARA_OUT : Outport  VectorParamsAs1DForOutWhenUnconnected=off
  SERIAL_OUT : Outport  Port=2  VectorParamsAs1DForOutWhenUnconnected=off
  wires:
  2BIT_SIPO/2(SERIAL_OUT) -> 2BIT_SIPO1/1(SERIAL_IN)
  2BIT_SIPO1/1(PARA_OUT) -> Vector Concatenate/1
  2BIT_SIPO/1(PARA_OUT) -> Vector Concatenate/2
  Vector Concatenate/1 -> PARA_OUT/1
  2BIT_SIPO1/2(SERIAL_OUT) -> SERIAL_OUT/1
  SERIAL_IN/1 -> 2BIT_SIPO/1(SERIAL_IN)

== system gm_rec_i2s/REC_I2S_FIFO/SIPO_32BIT_R1/Subsystem/SIPO_16BIT/SIPO_8BIT/SIPO_4BIT ==
  SERIAL_IN : Inport
  2BIT_SIPO : Subsystem
  2BIT_SIPO1 : Subsystem
  Vector Concatenate : Concatenate
  PARA_OUT : Outport  VectorParamsAs1DForOutWhenUnconnected=off
  SERIAL_OUT : Outport  Port=2  VectorParamsAs1DForOutWhenUnconnected=off
  wires:
  2BIT_SIPO/2(SERIAL_OUT) -> 2BIT_SIPO1/1(SERIAL_IN)
  2BIT_SIPO1/1(PARA_OUT) -> Vector Concatenate/1
  2BIT_SIPO/1(PARA_OUT) -> Vector Concatenate/2
  Vector Concatenate/1 -> PARA_OUT/1
  2BIT_SIPO1/2(SERIAL_OUT) -> SERIAL_OUT/1
  SERIAL_IN/1 -> 2BIT_SIPO/1(SERIAL_IN)

== system gm_rec_i2s/REC_I2S_FIFO/SIPO_32BIT_R1/Subsystem/SIPO_16BIT/SIPO_8BIT/SIPO_4BIT1 ==
  SERIAL_IN : Inport
  2BIT_SIPO : Subsystem
  2BIT_SIPO1 : Subsystem
  Vector Concatenate : Concatenate
  PARA_OUT : Outport  VectorParamsAs1DForOutWhenUnconnected=off
  SERIAL_OUT : Outport  Port=2  VectorParamsAs1DForOutWhenUnconnected=off
  wires:
  2BIT_SIPO/2(SERIAL_OUT) -> 2BIT_SIPO1/1(SERIAL_IN)
  2BIT_SIPO1/1(PARA_OUT) -> Vector Concatenate/1
  2BIT_SIPO/1(PARA_OUT) -> Vector Concatenate/2
  Vector Concatenate/1 -> PARA_OUT/1
  2BIT_SIPO1/2(SERIAL_OUT) -> SERIAL_OUT/1
  SERIAL_IN/1 -> 2BIT_SIPO/1(SERIAL_IN)
